simulink model "robot_varying_delay"  (R2022a)
settings: Solver=VariableStepAuto  StartTime=0.0  StopTime=sim_time  RelTol=1e-3
undefined symbols (not defined in the file): DiscIntNeverNeededParam, G, Kmpc, Kw, nmax, nmin, prediction_horizon, robot_continous_model, robot_vel, sampling_period, square_trajectory
libraries: simulink x2, dspsrcs4 x1
settings Model: Creator=mateus  LastModifiedBy=mateus

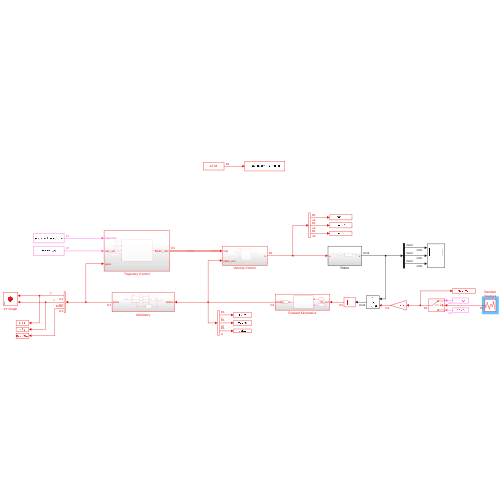
[thumbnail: Simulink's stored preview of the top-level diagram]
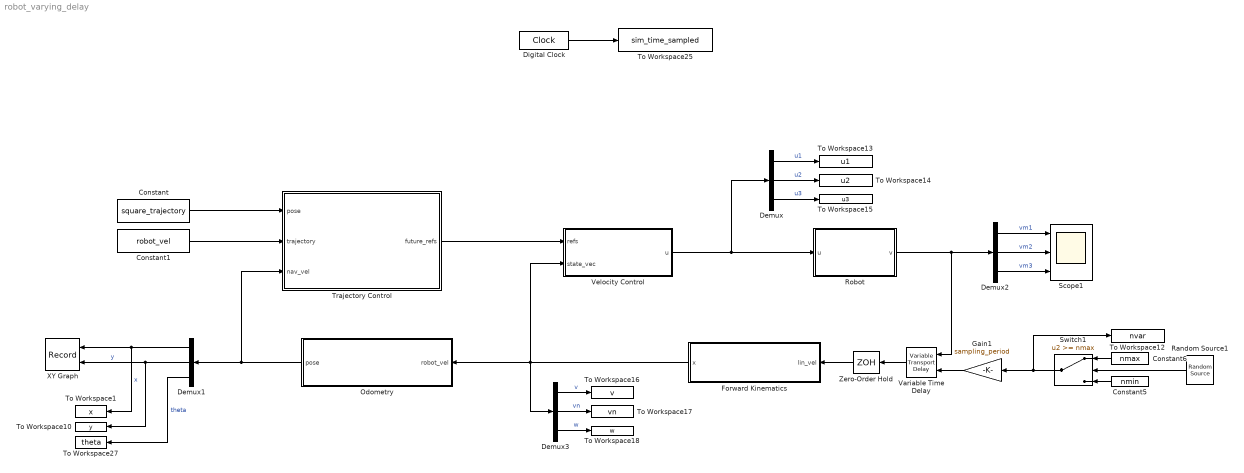
== system robot_varying_delay ==
  Constant : Constant  Value=square_trajectory  VectorParams1D=off
  Constant1 : Constant  Value=robot_vel  VectorParams1D=off
  Constant5 : Constant  Value=nmin
  Constant6 : Constant  Value=nmax
  Demux{,1..3} (4 alike) : Demux  Outputs=3
  Digital Clock : DigitalClock  SampleTime=sampling_period
  Forward Kinematics : Subsystem
  Gain1 : Gain  Gain=sampling_period
  Odometry : Subsystem
  Random Source1 : dspsrcs4/Random Source  SrcType=Uniform  NormMethod=Ziggurat  CltLength=12  MinVal=nmin  MaxVal=nmax+1  MeanVal=0  VarVal=1  RepMode=Specify seed  rawSeed=1  IsInherit=off  SampMode=Discrete  SampTime=sampling_period  SampFrame=1  DataType=Double  OutComplex=Real  OutputFrames=off
  Robot : Subsystem
  Scope1 : Scope  NumInputPorts=3
  Switch1 : Switch  Threshold=nmax  ZeroCross=off  SaturateOnIntegerOverflow=off  InputSameDT=off
  To Workspace1 : ToWorkspace  VariableName=x  SampleTime=-1
  To Workspace10 : ToWorkspace  VariableName=y  SampleTime=-1
  To Workspace12 : ToWorkspace  VariableName=nvar  SampleTime=-1
      settings: Save2DSignal=2-D array (concatenate along first dimension)
  To Workspace13 : ToWorkspace  VariableName=u1  SampleTime=-1
  To Workspace14 : ToWorkspace  VariableName=u2  SampleTime=-1
  To Workspace15 : ToWorkspace  VariableName=u3  SampleTime=-1
  To Workspace16 : ToWorkspace  VariableName=v  SampleTime=-1
      settings: Save2DSignal=2-D array (concatenate along first dimension)
  To Workspace17 : ToWorkspace  VariableName=vn  SampleTime=-1
      settings: Save2DSignal=2-D array (concatenate along first dimension)
  To Workspace18 : ToWorkspace  VariableName=w  SampleTime=-1
      settings: Save2DSignal=2-D array (concatenate along first dimension)
  To Workspace25 : ToWorkspace  VariableName=sim_time_sampled  SampleTime=sampling_period
      settings: Save2DSignal=2-D array (concatenate along first dimension)
  To Workspace27 : ToWorkspace  VariableName=theta  SampleTime=-1
  Trajectory Control : Subsystem
  Variable Time Delay : VariableTransportDelay  MaximumDelay=10  ZeroDelay=on
  Velocity Control : Subsystem
  XY Graph : Record  FileSettingsInternal="{\"entries\":[{\"content\":{\"excelSettings\":{\"content\":{},\"type\":\"Streamout.ExcelSettings\"}},\"type\":\"Streamout.FileSettingStorage\",\"uuid\":\"bc52e9b3-fcb7-4fd4-94df-b800869151ce\"}],\"packageUris\":[\"http://schema.mathworks.com/mf0/streamout_blocks/R2020a\"],\"version\":\"1.0\"}"  Layout=[1 1]  SignalsInternal="{\"entries\":[{\"content\":{\"signals\":[{\"content\":{\"blockPath\":[\"robot_varying_delay/XY Graph\"],\"channel\":[],\"dimensions\":[1],\"domain\":\"robot_varying_delay/XY Graph\",\"lineColor\":\"#a2142f\",\"plots\":[],\"port\":1,\"sid\":[\"\"],\"signalID\":12966,\"signalName\":\"x\"},\"type\":\"RecordBlkView.Signal\",\"uuid\":\"24f03dd4-a884-4c2e-9b9d-5f76e719e564\"},{\"content\":{\"blockPath\":[\"robot_varying_delay/XY Graph\"],\"channel\":[],\"dimensions\":[1],\"domain\":\"robot_varying_delay/XY Graph\",\"lineColor\":\"#139fff\",\"plots\":[],\"port\":2,\"sid\":[\"\"],\"signalID\":12970,\"signalName\":\"y\"},\"type\":\"RecordBlkView.Signal\",\"uuid\":\"8d5868cb-680d-4e95-affb-aafdb98a4794\"}]},\"type\":\"RecordBlkView.InputSignals\",\"uuid\":\"cfc90cf9-b9df-4466-9c7b-a72533a1d158\"}],\"packageUris\":[\"http://schema.mathworks.com/mf0/streamout_blocks/R2020a\"],\"version\":\"1.0\"}"  VisualizationBindings="{\"xyplotplugin\":{\"info\":[{\"series\":[],\"subplotID\":1}]}}"  CompatibilityTag=XY
  Zero-Order Hold : ZeroOrderHold  SampleTime=-1
  wires:
  Demux1/1 -> To Workspace1/1, XY Graph/1  "x"
  Demux1/2 -> To Workspace10/1, XY Graph/2  "y"
  Odometry/1(pose) -> Demux1/1, Trajectory Control/3(nav_vel)
  Constant1/1 -> Trajectory Control/2(trajectory)
  Trajectory Control/1(future_refs) -> Velocity Control/1(refs)
  Constant/1 -> Trajectory Control/1(pose)
  Demux/1 -> To Workspace13/1  "u1"
  Demux/2 -> To Workspace14/1  "u2"
  Demux/3 -> To Workspace15/1  "u3"
  Demux2/3 -> Scope1/3  "vm3"
  Demux2/2 -> Scope1/2  "vm2"
  Demux2/1 -> Scope1/1  "vm1"
  Forward Kinematics/1(x) -> Demux3/1, Velocity Control/2(state_vec), Odometry/1(robot_vel)
  Demux3/3 -> To Workspace18/1  "w"
  Demux3/2 -> To Workspace17/1  "vn"
  Demux3/1 -> To Workspace16/1  "v"
  Velocity Control/1(u) -> Robot/1(u), Demux/1
  Robot/1(v) -> Variable Time Delay/1, Demux2/1
  Zero-Order Hold/1 -> Forward Kinematics/1(lin_vel)
  Variable Time Delay/1 -> Zero-Order Hold/1
  Demux1/3 -> To Workspace27/1  "theta"
  Constant5/1 -> Switch1/3
  Constant6/1 -> Switch1/1
  Gain1/1 -> Variable Time Delay/2
  Random Source1/1 -> Switch1/2
  Switch1/1 -> To Workspace12/1, Gain1/1
  Digital Clock/1 -> To Workspace25/1

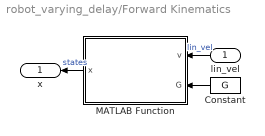
== system robot_varying_delay/Forward Kinematics ==
  lin_vel : Inport
  Constant : Constant  Value=G  VectorParams1D=off
  MATLAB Function : MATLAB Function  TreatAsAtomicUnit=on
  x : Outport
  wires:
  Constant/1 -> MATLAB Function/2(G)
  lin_vel/1 -> MATLAB Function/1(v)  "lin_vel"
  MATLAB Function/1(x) -> x/1  "states"

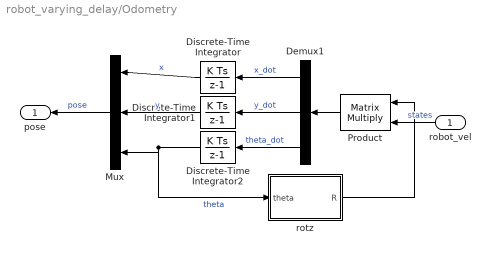
== system robot_varying_delay/Odometry ==
  robot_vel : Inport
  Demux1 : Demux  Outputs=3
  Discrete-Time Integrator : DiscreteIntegrator  SampleTime=sampling_period  ICPrevOutput=DiscIntNeverNeededParam  ICPrevScaledInput=DiscIntNeverNeededParam
  Discrete-Time Integrator1 : DiscreteIntegrator  SampleTime=sampling_period  ICPrevOutput=DiscIntNeverNeededParam  ICPrevScaledInput=DiscIntNeverNeededParam
  Discrete-Time Integrator2 : DiscreteIntegrator  SampleTime=sampling_period  ICPrevOutput=DiscIntNeverNeededParam  ICPrevScaledInput=DiscIntNeverNeededParam
  Mux : Mux  Inputs=3
  Product : Product  Multiplication=Matrix(*)
  rotz : MATLAB Function  TreatAsAtomicUnit=on  SystemSampleTime=sampling_period
  pose : Outport
  wires:
  robot_vel/1 -> Product/2  "states"
  Discrete-Time Integrator1/1 -> Mux/2  "y"
  Demux1/1 -> Discrete-Time Integrator/1  "x_dot"
  Demux1/3 -> Discrete-Time Integrator2/1  "theta_dot"
  rotz/1(R) -> Product/1
  Product/1 -> Demux1/1
  Demux1/2 -> Discrete-Time Integrator1/1  "y_dot"
  Discrete-Time Integrator2/1 -> Mux/3, rotz/1(theta)  "theta"
  Discrete-Time Integrator/1 -> Mux/1  "x"
  Mux/1 -> pose/1  "pose"

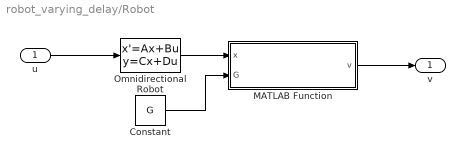
== system robot_varying_delay/Robot ==
  u : Inport
  Constant : Constant  Value=G  VectorParams1D=off
  MATLAB Function : MATLAB Function  TreatAsAtomicUnit=on
  Omnidirectional Robot : StateSpace  A=robot_continous_model.A  B=robot_continous_model.B  C=robot_continous_model.C  D=robot_continous_model.D  InitialCondition=[0; 0; 0]  ContinuousStateAttributes=states
  v : Outport
  wires:
  Constant/1 -> MATLAB Function/2(G)
  Omnidirectional Robot/1 -> MATLAB Function/1(x)
  MATLAB Function/1(v) -> v/1
  u/1 -> Omnidirectional Robot/1

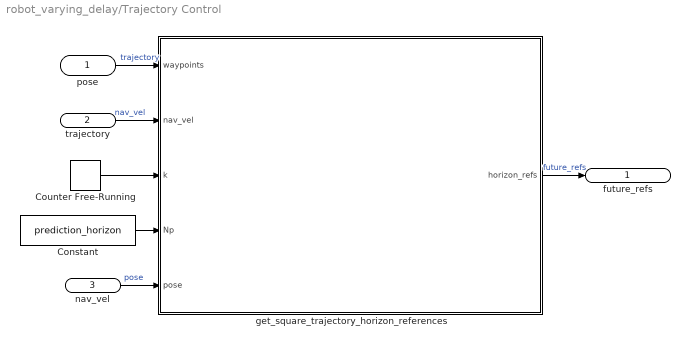
== system robot_varying_delay/Trajectory Control ==
  pose : Inport
  trajectory : Inport  Port=2  SampleTime=sampling_period
  nav_vel : Inport  Port=3
  Constant : Constant  Value=prediction_horizon  VectorParams1D=off
  Counter Free-Running : simulink/Sources/Counter Free-Running  NumBits=16  tsamp=sampling_period
  get_square_trajectory_horizon_references : MATLAB Function  TreatAsAtomicUnit=on  SystemSampleTime=sampling_period
  future_refs : Outport
  wires:
  Constant/1 -> get_square_trajectory_horizon_references/4(Np)
  Counter Free-Running/1 -> get_square_trajectory_horizon_references/3(k)
  get_square_trajectory_horizon_references/1(horizon_refs) -> future_refs/1  "future_refs"
  trajectory/1 -> get_square_trajectory_horizon_references/2(nav_vel)  "nav_vel"
  pose/1 -> get_square_trajectory_horizon_references/1(waypoints)  "trajectory"
  nav_vel/1 -> get_square_trajectory_horizon_references/5(pose)  "pose"

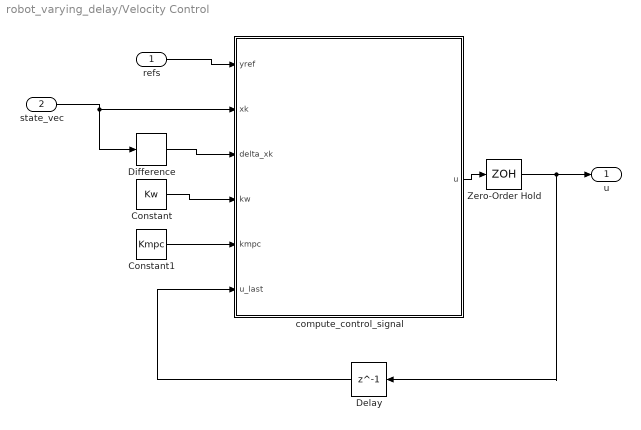
== system robot_varying_delay/Velocity Control ==
  refs : Inport  SampleTime=sampling_period
  state_vec : Inport  Port=2
  Constant : Constant  Value=Kw  VectorParams1D=off
  Constant1 : Constant  Value=Kmpc  VectorParams1D=off
  Delay : Delay  DelayLength=1  InitialCondition=0
  Difference : simulink/Discrete/Difference  ICPrevInput=0.0  OutMin=[]  OutMax=[]  OutDataType=fixdt(1, 16)  OutScaling=2^-10  DoSatur=off
  Zero-Order Hold : ZeroOrderHold  SampleTime=sampling_period
  compute_control_signal : MATLAB Function  TreatAsAtomicUnit=on
  u : Outport
  wires:
  compute_control_signal/1(u) -> Zero-Order Hold/1
  state_vec/1 -> compute_control_signal/2(xk), Difference/1
  Difference/1 -> compute_control_signal/3(delta_xk)
  refs/1 -> compute_control_signal/1(yref)
  Constant/1 -> compute_control_signal/4(kw)
  Constant1/1 -> compute_control_signal/5(kmpc)
  Delay/1 -> compute_control_signal/6(u_last)
  Zero-Order Hold/1 -> Delay/1, u/1

== matlab function robot_varying_delay/Forward Kinematics/MATLAB Function ==
  data: v input; x output; G input
function x = forward_kinematics(v, G)
  x = G\v;
end

== matlab function robot_varying_delay/Robot/MATLAB Function ==
  data: x input; v output; G input
function v = inverse_kinematics(x, G)
%INVERSE_KINEMATICS Return the linear velocities given the state vector
  v = G*x;
end

== matlab function robot_varying_delay/Odometry/rotz ==
  data: theta input; R output
function R = rotz(theta)
    %ROTZ Get the rotation matrix around z axis given the angle theta
    R = [cos(theta) sin(theta) 0; -sin(theta) cos(theta) 0; 0 0 1]';
end

== matlab function robot_varying_delay/Trajectory Control/get_square_trajectory_horizon_references ==
  data: waypoints input; nav_vel input; k input; Np input; horizon_refs output size=[prediction_horizon*3 1] [0..10]; pose input
function horizon_refs = get_square_trajectory_horizon_references(waypoints, nav_vel, k, Np, pose)
    % Future references must be in Y = [yr(k) yr(k+1) ... yr(k+N-1)]
    horizon_refs = zeros(Np*3,1);
 
    k=k+1;

    x=pose(1);
    y=pose(2);
    theta=pose(3);
    tol = 0.01;

    if (k > length(waypoints))
        return
    end

    i=1;
    for j=k:k+Np-1
        Rz = [cos(theta) sin(theta) 0; -sin(theta) cos(theta) 0; 0 0 1];

        if j > length(waypoints)
            x_ref = waypoints(1,end);
            y_ref = waypoints(2,end);
            theta_ref = waypoints(3,end);
        else
            x_ref = waypoints(1,j);
            y_ref = waypoints(2,j);
            theta_ref = waypoints(3,j);
        end
 
        phi = atan2(y_ref-y, x_ref-x);  % atan2(yr(k + j|k) - yr(k), xr(k + j|k) − xr(k))
        temp_vec = [nav_vel*cos(phi) nav_vel*sin(phi) theta_ref-theta]';
        temp_vec = Rz*temp_vec;
        horizon_refs(i:i+2,1) = temp_vec;
        i=i+3;
    end
end

== matlab function robot_varying_delay/Velocity Control/compute_control_signal ==
  data: yref input; u output; xk input; delta_xk input; kw input; kmpc input; u_last input
function u = compute_control_signal(yref, xk, delta_xk, kw, kmpc, u_last)
    ksi = [delta_xk; xk];    % In this case, y[k] is the state vector due C = I
    delta_u = kw*yref - kmpc*ksi;
    u = delta_u(1:3,1) + u_last;
end
